simulink model "lab1"  (R2020a)
settings: Solver=VariableStepAuto  StartTime=0.0  StopTime=10.0  RelTol=1e-3
libraries: simulink_extras x1, simulink x1
settings Model: Creator=root  LastModifiedBy=root

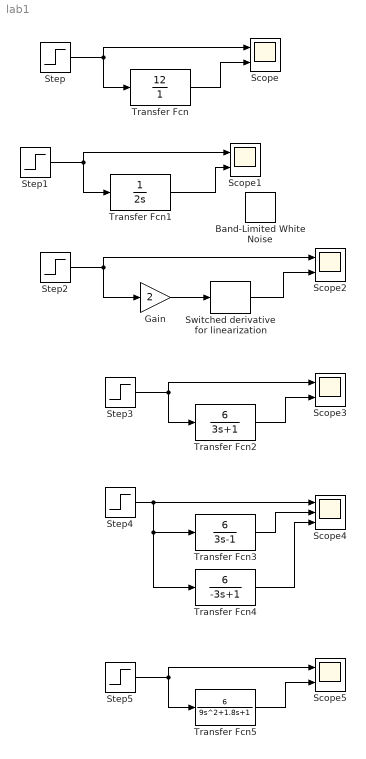
== system lab1 ==
  Gain : Gain  Gain=2
  Scope{,1..3,5} (5 alike) : Scope  NumInputPorts=2
  Scope4 : Scope  NumInputPorts=3
  Step{,1..5} (6 alike) : Step  SampleTime=0
  Switched derivative for linearization : simulink_extras/Linearization/Switched derivative for linearization  switchVal=1  derivConst=1
      settings: SourceProductBaseCode=SL
  Transfer Fcn : TransferFcn  Numerator=[12]  Denominator=[1]
  Transfer Fcn1 : TransferFcn  Denominator=[2, 0]
  Transfer Fcn2 : TransferFcn  Numerator=[6]  Denominator=[3 1]
  Transfer Fcn3 : TransferFcn  Numerator=[6]  Denominator=[3 -1]
  Transfer Fcn4 : TransferFcn  Numerator=[6]  Denominator=[-3 1]
  Transfer Fcn5 : TransferFcn  Numerator=[6]  Denominator=[9 1.8 1]
  Band-Limited White Noise : simulink/Sources/Band-Limited White Noise  IOType=siggen  Cov=[0.1]  Ts=0.1  seed=[23341]
  wires:
  Step/1 -> Transfer Fcn/1, Scope/1
  Transfer Fcn/1 -> Scope/2
  Transfer Fcn1/1 -> Scope1/2
  Step1/1 -> Transfer Fcn1/1, Scope1/1
  Step2/1 -> Gain/1, Scope2/1
  Gain/1 -> Switched derivative for linearization/1
  Switched derivative for linearization/1 -> Scope2/2
  Transfer Fcn2/1 -> Scope3/2
  Step3/1 -> Transfer Fcn2/1, Scope3/1
  Step4/1 -> Transfer Fcn4/1, Transfer Fcn3/1, Scope4/1
  Transfer Fcn3/1 -> Scope4/2
  Transfer Fcn4/1 -> Scope4/3
  Step5/1 -> Transfer Fcn5/1, Scope5/1
  Transfer Fcn5/1 -> Scope5/2
